simulink model "LAB1_ThermalProcessSimulation"  (R2025b)
settings: Solver=VariableStepAuto  StartTime=0.0  StopTime=1000  RelTol=1e-3
settings Model: Creator=Wingshingsho  LastModifiedBy=Wingshingsho

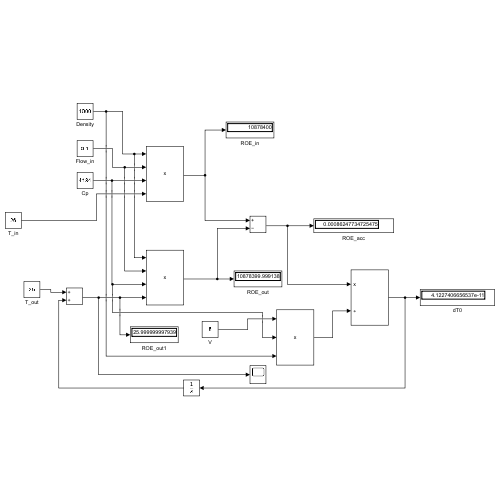
[thumbnail: Simulink's stored preview of the top-level diagram]
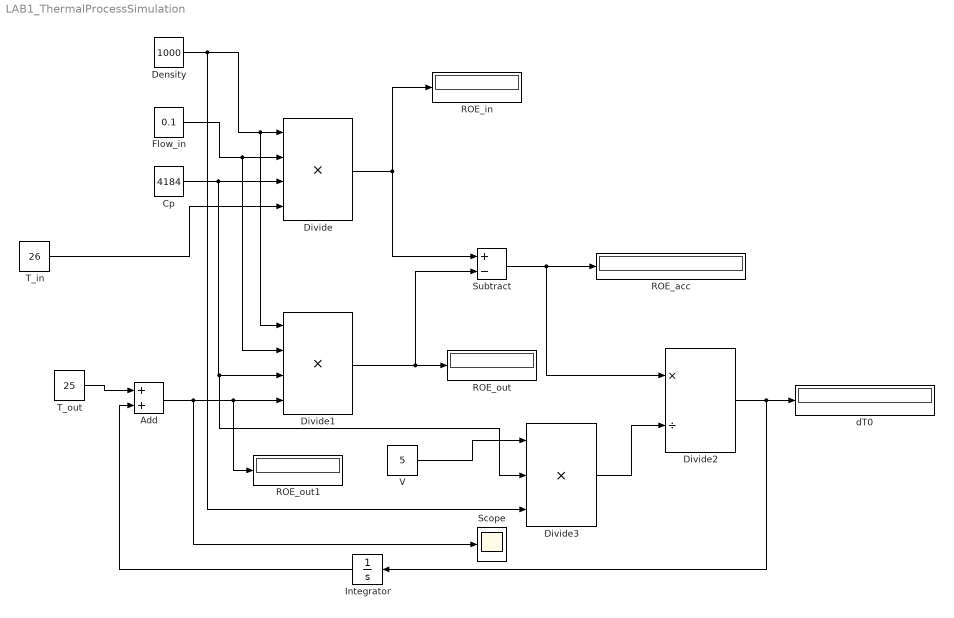
== system LAB1_ThermalProcessSimulation ==
  Add : Sum
  Cp : Constant  Value=4184
  Density : Constant  Value=1000
  Divide : Product  Inputs=****
  Divide1 : Product  Inputs=****
  Divide2 : Product  Inputs=*/
  Divide3 : Product  Inputs=***
  Flow_in : Constant  Value=0.1
  Integrator : Integrator
  ROE_acc : Display
  ROE_in : Display
  ROE_out : Display
  ROE_out1 : Display
  Scope : Scope
      settings: ActiveDisplayYMinimum=24.509157819481782  ActiveDisplayYMaximum=29.417579624663958
  Subtract : Sum  Inputs=+-
  T_in : Constant  Value=26
  T_out : Constant  Value=25
  V : Constant  Value=5
  dT0 : Display
  wires:
  Density/1 -> Divide1/1, Divide/1, Divide3/3
  Flow_in/1 -> Divide1/2, Divide/2
  Cp/1 -> Divide3/2, Divide1/3, Divide/3
  Divide/1 -> Subtract/1, ROE_in/1
  Divide1/1 -> Subtract/2, ROE_out/1
  Subtract/1 -> Divide2/1, ROE_acc/1
  V/1 -> Divide3/1
  Divide3/1 -> Divide2/2
  Divide2/1 -> Integrator/1, dT0/1
  Integrator/1 -> Add/2
  T_out/1 -> Add/1
  Add/1 -> Scope/1, ROE_out1/1, Divide1/4
  T_in/1 -> Divide/4
